simulink model "VehiclePlant"  (R2026a)
settings: configuration reference "standardSILConfiguraitonParams" (kept outside this file)
values from neighbouring files (symbols this model uses):
  vehicleParams = evalin('base', 'vehicleParams')    [testVehicleSIL.m]
settings Model: Creator=GTAR  LastModifiedBy=Edison Altamirano
settings ConfigSetRef: SourceName=standardSILConfiguraitonParams  SourceLocation=Base Workspace

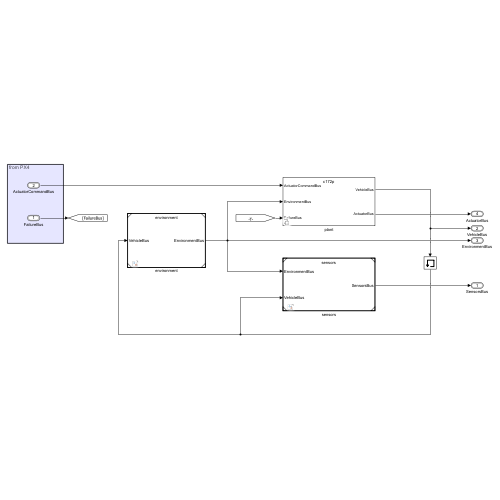
[thumbnail: Simulink's stored preview of the top-level diagram]
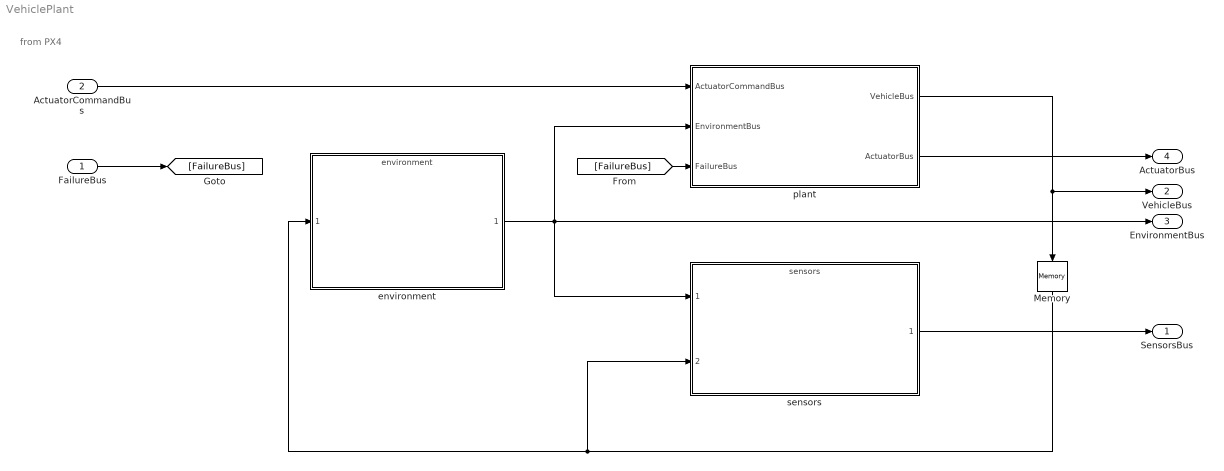
== system VehiclePlant ==
  note: from PX4
  FailureBus : Inport  OutDataTypeStr=Bus: FailureBus
  ActuatorCommandBus : Inport  Port=2  OutDataTypeStr=Bus: ActuatorCommandBus  LockScale=on
  Memory : Memory
  environment : ModelReference  ModelNameDialog=environment.slx  SimulationMode=Normal  ModelReferenceVersion=1.14
  plant : Subsystem  Variant=on
  sensors : ModelReference  ModelNameDialog=sensors.slx  SimulationMode=Normal  ModelReferenceVersion=5.1
  SensorsBus : Outport  OutDataTypeStr=Bus: SensorsBus
  VehicleBus : Outport  Port=2  OutDataTypeStr=Bus: VehicleBus
  EnvironmentBus : Outport  Port=3  OutDataTypeStr=Bus: EnvironmentBus
  ActuatorBus : Outport  Port=4  OutDataTypeStr=Bus: ActuatorBus
  wires:
  sensors/1 -> SensorsBus/1
  ActuatorCommandBus/1 -> plant/1(ActuatorCommandBus)
  environment/1 -> sensors/1, EnvironmentBus/1, plant/2(EnvironmentBus)
  Memory/1 -> sensors/2, environment/1
  plant/1(VehicleBus) -> VehicleBus/1, Memory/1
  FailureBus/1 -> [FailureBus]
  [FailureBus] -> plant/3(FailureBus)
  plant/2(ActuatorBus) -> ActuatorBus/1

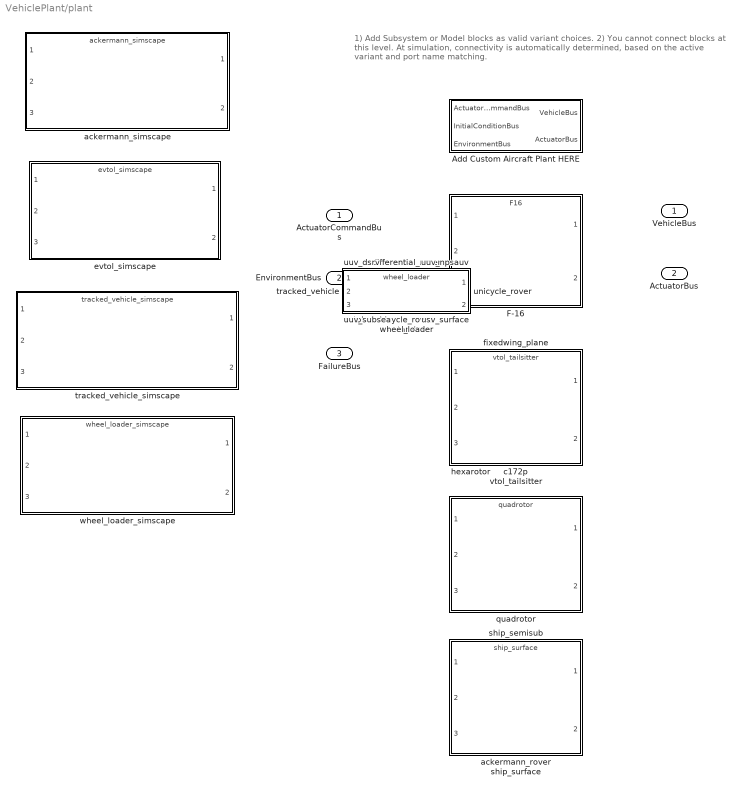
== system VehiclePlant/plant ==
  note: 1) Add Subsystem or Model blocks as valid variant choices.
      | 2) You cannot connect blocks at this level. At simulation, connectivity is automatically
      | determined, based on the active variant and port name matching.
  ActuatorCommandBus : Inport  OutDataTypeStr=Bus: ActuatorCommandBus  LockScale=on
  EnvironmentBus : Inport  Port=2  OutDataTypeStr=Bus: EnvironmentBus
  FailureBus : Inport  Port=3  OutDataTypeStr=Bus: FailureBus
  Add Custom Aircraft Plant HERE : Subsystem  VariantControl="strcmpi(vehicleParams.type ,\"Custom\")"
  F-16 : ModelReference  ModelNameDialog=F16.slx  VariantControl="strcmpi(vehicleParams.baseVehicleType ,\"F-16\")"  ModelReferenceVersion=1.120
  ackermann_rover : ModelReference  ModelNameDialog=ackermann_rover  SimulationMode=Normal  VariantControl="strcmpi(vehicleParams.type ,\"ackermann_rover\")"  ModelReferenceVersion=5.1
  ackermann_simscape : ModelReference  ModelNameDialog=ackermann_simscape  VariantControl="strcmpi(vehicleParams.type ,\"ackermann_simscape\")"  ModelReferenceVersion=5.0
  bicycle_rover : ModelReference  ModelNameDialog=bicycle_rover  SimulationMode=Normal  VariantControl="strcmpi(vehicleParams.type ,\"bicycle_rover\")"  ModelReferenceVersion=1.56
  c172p : ModelReference  ModelNameDialog=c172p  SimulationMode=Normal  VariantControl="strcmpi(vehicleParams.type ,\"c172p\")"  ModelReferenceVersion=5.0
  differential_rover : ModelReference  ModelNameDialog=differential_rover  SimulationMode=Normal  VariantControl="strcmpi(vehicleParams.type ,\"differential_rover\")"  ModelReferenceVersion=1.56
  evtol : ModelReference  ModelNameDialog=evtol  SimulationMode=Normal  VariantControl="strcmpi(vehicleParams.type ,\"evtol\")"  ModelReferenceVersion=1.56
  evtol_simscape : ModelReference  ModelNameDialog=evtol_simscape  VariantControl="strcmpi(vehicleParams.type ,\"evtol_simscape\")"  ModelReferenceVersion=5.0
  fixedwing_plane : ModelReference  ModelNameDialog=fixedwing_plane.slx  SimulationMode=Normal  VariantControl="strcmpi(vehicleParams.type ,\"fixedwing_plane\")"  ModelReferenceVersion=5.0
  hexarotor : ModelReference  ModelNameDialog=hexarotor.slx  SimulationMode=Normal  VariantControl="strcmpi(vehicleParams.type ,\"hexarotor\")"  ModelReferenceVersion=1.56
  octarotor : ModelReference  ModelNameDialog=octarotor  SimulationMode=Normal  VariantControl="strcmpi(vehicleParams.type ,\"octarotor\")"  ModelReferenceVersion=1.56
  quadrotor : ModelReference  ModelNameDialog=quadrotor  SimulationMode=Normal  VariantControl="strcmpi(vehicleParams.type ,\"quadrotor\")"  ModelReferenceVersion=1.56
  ship_semisub : ModelReference  ModelNameDialog=ship_semisub.slx  SimulationMode=Normal  VariantControl="strcmpi(vehicleParams.type ,\"ship_semisub\")"  ModelReferenceVersion=5.4
  ship_surface : ModelReference  ModelNameDialog=ship_surface.slx  SimulationMode=Normal  VariantControl="strcmpi(vehicleParams.type ,\"ship_surface\")"  ModelReferenceVersion=5.3
  tracked_vehicle : ModelReference  ModelNameDialog=tracked_vehicle  SimulationMode=Normal  VariantControl="strcmpi(vehicleParams.type ,\"tracked_vehicle\")"  ModelReferenceVersion=1.56
  tracked_vehicle_simscape : ModelReference  ModelNameDialog=tracked_vehicle_simscape  VariantControl="strcmpi(vehicleParams.type ,\"tracked_vehicle_simscape\")"  ModelReferenceVersion=5.0
  unicycle_rover : ModelReference  ModelNameDialog=unicycle_rover  SimulationMode=Normal  VariantControl="strcmpi(vehicleParams.type ,\"unicycle_rover\")"  ModelReferenceVersion=1.56
  usv_surface : ModelReference  ModelNameDialog=usv_surface  SimulationMode=Normal  VariantControl="strcmpi(vehicleParams.type ,\"usv_surface\")"  ModelReferenceVersion=1.56
  uuv_dsrv : ModelReference  ModelNameDialog=uuv_dsrv.slx  SimulationMode=Normal  VariantControl="strcmpi(vehicleParams.type ,\"uuv_dsrv\")"  ModelReferenceVersion=5.2
  uuv_npsauv : ModelReference  ModelNameDialog=uuv_npsauv.slx  SimulationMode=Normal  VariantControl="strcmpi(vehicleParams.type ,\"uuv_npsauv\")"  ModelReferenceVersion=5.3
  uuv_subsea : ModelReference  ModelNameDialog=uuv_subsea  SimulationMode=Normal  VariantControl="strcmpi(vehicleParams.type ,\"uuv_subsea\")"  ModelReferenceVersion=5.2
  vtol_tailsitter : ModelReference  ModelNameDialog=vtol_tailsitter.slx  SimulationMode=Normal  VariantControl="strcmpi(vehicleParams.type ,\"vtol_tailsitter\")"  ModelReferenceVersion=1.56
  wheel_loader : ModelReference  ModelNameDialog=wheel_loader  SimulationMode=Normal  VariantControl="strcmpi(vehicleParams.type ,\"wheel_loader\")"  ModelReferenceVersion=1.56
  wheel_loader_simscape : ModelReference  ModelNameDialog=wheel_loader_simscape  VariantControl="strcmpi(vehicleParams.type ,\"wheel_loader_simscape\")"  ModelReferenceVersion=5.0
  VehicleBus : Outport
  ActuatorBus : Outport  Port=2

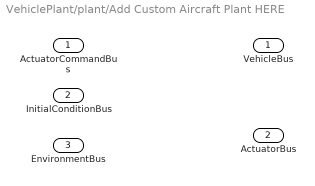
== system VehiclePlant/plant/Add Custom Aircraft Plant HERE ==
  ActuatorCommandBus : Inport
  InitialConditionBus : Inport  Port=2
  EnvironmentBus : Inport  Port=3
  VehicleBus : Outport
  ActuatorBus : Outport  Port=2  OutDataTypeStr=Bus: ActuatorBus
